simulink model "manyUnitDelay2_20160126_142201"  (R2014a)
settings: Solver=FixedStepDiscrete  StartTime=0.0  StopTime=10.0  FixedStep=1  RelTol=1e-3
settings Model: Creator=yoshi12  LastModifiedBy=yoshi12

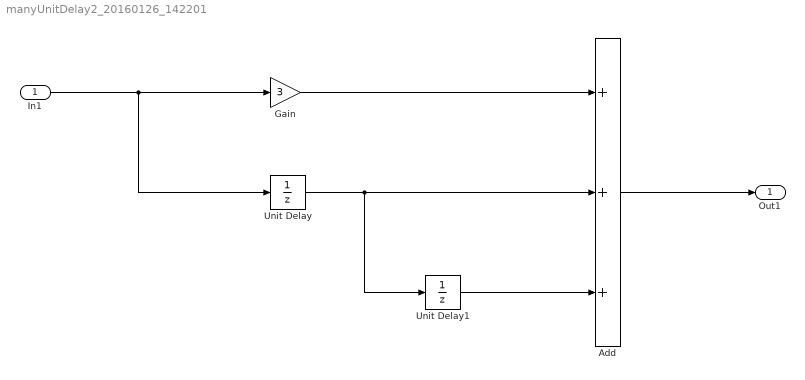
== system manyUnitDelay2_20160126_142201 ==
  In1 : Inport
  Add : Sum  Inputs=+++
  Gain : Gain  Gain=3
  Unit Delay : UnitDelay  SampleTime=-1
  Unit Delay1 : UnitDelay  SampleTime=-1
  Out1 : Outport
  wires:
  In1/1 -> Unit Delay/1, Gain/1
  Unit Delay/1 -> Unit Delay1/1, Add/2
  Gain/1 -> Add/1
  Unit Delay1/1 -> Add/3
  Add/1 -> Out1/1
